simulink model "tank_model"  (R2019b)
settings: Solver=VariableStepAuto  StartTime=0.0  StopTime=10.0  RelTol=1e-3
InitFcn:
  | load('parameters.mat')
  | load('equibrium.mat')
  | load('linearized_matrix.mat')
values from neighbouring files (symbols this model uses):
  A = [-k1/(2*xe(1)^(1/2)), 0 ... (first row only)    [linearization.m]    (also in workspace.mat = [-0.0391932075235  0; 0.0391932075235  -0.0381972328031])
  alpha1 = 0.055    [equibrium.m]    (also in parameters.mat; workspace.mat)
  alpha2 = 0.059    [equibrium.m]    (also in parameters.mat; workspace.mat)
  b = [gamma1/(2*(beta1 + gamma1*ue(1))^(1/2)); 0]    [linearization.m]    (also in workspace.mat = [0.936765947069 0])
  beta1 = -3.077    [equibrium.m]    (also in parameters.mat; workspace.mat)
  beta2 = -3.246    [equibrium.m]    (also in parameters.mat; workspace.mat)
  gamma1 = 3.551    [equibrium.m]    (also in parameters.mat; workspace.mat)
  gamma2 = 3.610    (= 3.61)    [equibrium.m]    (also in parameters.mat; workspace.mat)
  k1 = 0.391    [equibrium.m]    (also in parameters.mat; workspace.mat)
  k2 = 0.386    [equibrium.m]    (also in parameters.mat; workspace.mat)
  ue = [ue1; ue2]    [equibrium.m]    (also in equibrium.mat = [1.87816229294 0]; workspace.mat = [1.87816229294 0])
  xe = [xe1; xe2]    [equibrium.m]    (also in equibrium.mat = [24.8812336392 25.53]; workspace.mat = [24.8812336392 25.53])
settings Model: Creator=tongk  LastModifiedBy=tongk

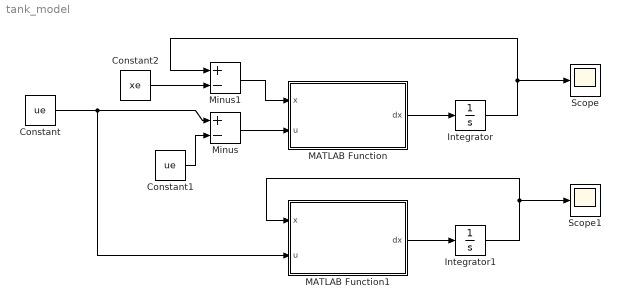
== system tank_model ==
  Constant : Constant  Value=ue
  Constant1 : Constant  Value=ue
  Constant2 : Constant  Value=xe
  Integrator : Integrator  InitialCondition=[0; 0]
  Integrator1 : Integrator  InitialCondition=xe
  MATLAB Function : MATLAB Function  TreatAsAtomicUnit=on
  MATLAB Function1 : MATLAB Function  TreatAsAtomicUnit=on
  Minus : Sum  Inputs=+-
  Minus1 : Sum  Inputs=+-
  Scope : Scope
  Scope1 : Scope
  wires:
  MATLAB Function/1(dx) -> Integrator/1
  Integrator/1 -> Minus1/1, Scope/1
  Constant/1 -> Minus/1, MATLAB Function1/2(u)
  Minus/1 -> MATLAB Function/2(u)
  Constant1/1 -> Minus/2
  MATLAB Function1/1(dx) -> Integrator1/1
  Integrator1/1 -> Scope1/1, MATLAB Function1/1(x)
  Minus1/1 -> MATLAB Function/1(x)
  Constant2/1 -> Minus1/2

== matlab function tank_model/MATLAB Function1 ==
  data: x input; dx output; u input; beta1 parameter; beta2 parameter; gamma1 parameter; gamma2 parameter; k1 parameter; k2 parameter; alpha1 parameter; alpha2 parameter
function dx = non_linear_model(x, u, beta1, beta2, gamma1, gamma2, k1, k2, alpha1, alpha2)

    function z=zp(u, i)
        if i == 1
            if beta1 + gamma1 * u > 0
                z = alpha1 + sqrt(beta1 + gamma1 * u);
            else
                z = 0;
            end
        elseif i == 2
            if beta2 + gamma2 * u > 0
                z = alpha2 + sqrt(beta2 + gamma2 * u);
            else
                z = 0;
            end
        end

    end
    
dx = [0; 0];      
zp1 = zp(u(1), 1);
zp2 = zp(u(2), 2);
dx = [-k1 * sqrt(x(1)) + zp1; -k2 * sqrt(x(2)) + k1 * sqrt(x(1)) + zp2];

end

== matlab function tank_model/MATLAB Function ==
  data: x input; dx output; u input; b parameter; A parameter
function dx = linear_model(x, u, b, A)
dx = [0; 0];
dx = A * x + b * u(1);

end
